simulink model "simulazione_sistema_osservatore_con_disturbo"  (R2019b)
settings: Solver=VariableStepAuto  StartTime=0.0  StopTime=50  RelTol=1e-3
values from neighbouring files (symbols this model uses):
  A = [0 0 1 0;0 0 0 1;-k/m1 k/m1 -c/m1 c/m1;k/m2 -k/m2 c/m2 -c/m2]    [ValoriCaso1.m]    (also in ValoriCaso2.m; ValoriCaso3.m; ValoriCaso4.m; ValoriCaso5.m)
  B = [0;0;1/m1;0]    [ValoriCaso1.m]    (also in ValoriCaso2.m; ValoriCaso3.m; ValoriCaso4.m; ValoriCaso5.m)
  C = [1 0 0 0]    [ValoriCaso1.m]    (also in ValoriCaso2.m; ValoriCaso3.m; ValoriCaso4.m; ValoriCaso5.m)
  M = [0;0;0;1/m2]    [ValoriCaso1.m]    (also in ValoriCaso2.m; ValoriCaso3.m; ValoriCaso4.m; ValoriCaso5.m)
  mat_f = A-(V*C)    [CreazioneOsservatore.m]
  V = -(Fd')    [CreazioneOsservatore.m]
settings Model: Creator=sugam  LastModifiedBy=sugam

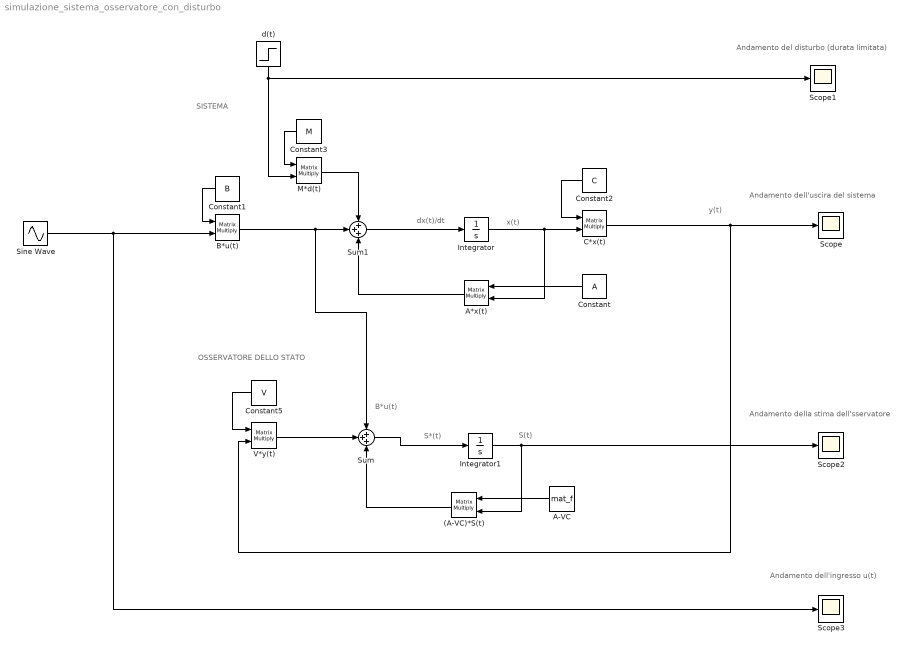
== system simulazione_sistema_osservatore_con_disturbo ==
  note: Andamento dell'ingresso u(t)
  note: Andamento della stima dell'sservatore
  note: OSSERVATORE DELLO STATO
  note: B*u(t)
  note: S(t)
  note: S*(t)
  note: SISTEMA
  note: Andamento dell'uscira del sistema
  note: Andamento del disturbo (durata limitata)
  note: y(t)
  note: x(t)
  note: dx(t)/dt
  (A-VC)*S(t) : Product  Multiplication=Matrix(*)
  A*x(t) : Product  Multiplication=Matrix(*)
  A-VC : Constant  Value=mat_f  VectorParams1D=off  SampleTime=0
  B*u(t) : Product  Multiplication=Matrix(*)
  C*x(t) : Product  Multiplication=Matrix(*)
  Constant : Constant  Value=A  VectorParams1D=off  SampleTime=0
  Constant1 : Constant  Value=B  VectorParams1D=off  SampleTime=0
  Constant2 : Constant  Value=C  VectorParams1D=off  SampleTime=0
  Constant3 : Constant  Value=M  VectorParams1D=off  SampleTime=0
  Constant5 : Constant  Value=V  VectorParams1D=off  SampleTime=0
  Integrator : Integrator
  Integrator1 : Integrator
  M*d(t) : Product  Multiplication=Matrix(*)
  Scope{,1..3} (4 alike) : Scope
  Sine Wave : Sin  Amplitude=5  Frequency=2  SampleTime=0
  Sum : Sum  Inputs=+++
  Sum1 : Sum  Inputs=+++
  V*y(t) : Product  Multiplication=Matrix(*)
  d(t) : Step  Time=10  Before=5  After=0  SampleTime=0  VectorParams1D=off
  wires:
  Constant1/1 -> B*u(t)/1
  Sum1/1 -> Integrator/1
  Integrator/1 -> A*x(t)/2, C*x(t)/2
  Constant2/1 -> C*x(t)/1
  C*x(t)/1 -> V*y(t)/2, Scope/1
  Constant3/1 -> M*d(t)/1
  B*u(t)/1 -> Sum1/2, Sum/1
  Constant/1 -> A*x(t)/1
  d(t)/1 -> Scope1/1, M*d(t)/2
  Constant5/1 -> V*y(t)/1
  V*y(t)/1 -> Sum/2
  Sum/1 -> Integrator1/1
  Integrator1/1 -> (A-VC)*S(t)/2, Scope2/1
  A-VC/1 -> (A-VC)*S(t)/1
  (A-VC)*S(t)/1 -> Sum/3
  Sine Wave/1 -> Scope3/1, B*u(t)/2
  M*d(t)/1 -> Sum1/1
  A*x(t)/1 -> Sum1/3
